simulink model "PROVA__14_10"  (R2020b)
settings: Solver=FixedStepDiscrete  StartTime=0.0  StopTime=Inf  FixedStep=0.02  RelTol=1e-3  EnableMultiTasking=on
undefined symbols (not defined in the file or in its folder): attuatore_Amax, attuatore_Amin, attuatore_Emax, attuatore_Emin, attuatore_Rmax, attuatore_Rmin, attuatore_Tmax, attuatore_Tmin, DiscIntNeverNeededParam, interventoA_05, interventoA_1, interventoE_05, interventoE_1, interventoT, inv_A, inv_comp_h, inv_E, inv_R, inv_T, K_AW_B_AP_quota, K_AW_B_becc, K_AW_B_imb, K_AW_B_roll, K_imb_inv, Kd_h_app, Kd_h_flare, Ki_AP_quota_select, Ki_AP_rotta, Ki_AP_vel, Ki_becch, Ki_h_app, Ki_h_cruise, Ki_h_flare, Ki_roll, Kp_AP_quota_hold_h, Kp_AP_quota_hold_l, Kp_AP_quota_select, Kp_AP_rotta, Kp_AP_vel, Kp_becch, Kp_comp_h, Kp_h_app_max, Kp_h_app_min, Kp_h_cruise, Kp_h_flare, Kp_imb, Kp_p, Kp_q, Kp_roll, Kp_Rotta_ATO, Newton, phi_max, phi_min, Raphson, safe_phi, safe_V, t_AP, theta_max, theta_min, time_alarm_SAFE ... (+5)
libraries: simulink_extras x34, arduinolib x24, pid_lib x8, simulink x3, dspsigops x3, svdutilitieslib x3, aerolibtransform2sys x2, aerolibtransform2 x2
(part 4 of 7)

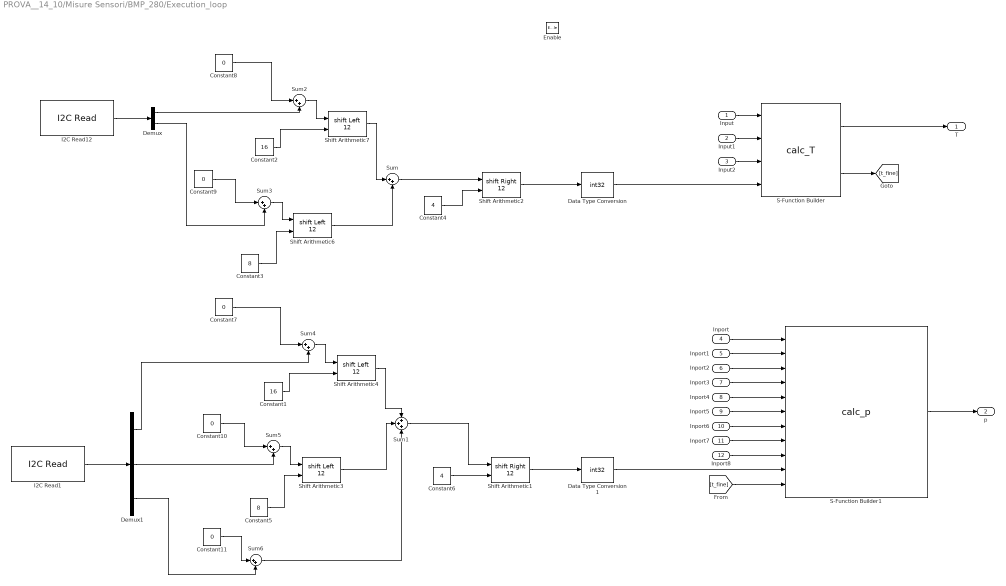
== system PROVA__14_10/Misure Sensori/BMP_280/Execution_loop ==
  Input : Inport
  Input1 : Inport  Port=2
  Input2 : Inport  Port=3
  Inport : Inport  Port=4
  Inport1 : Inport  Port=5
  Inport2 : Inport  Port=6
  Inport3 : Inport  Port=7
  Inport4 : Inport  Port=8
  Inport5 : Inport  Port=9
  Inport6 : Inport  Port=10
  Inport7 : Inport  Port=11
  Inport8 : Inport  Port=12
  Enable : EnablePort
  Constant1 : Constant  Value=16
  Constant{7..11} (5 alike) : Constant  Value=0  OutDataTypeStr=uint32
  Constant2 : Constant  Value=16
  Constant3 : Constant  Value=8
  Constant4 : Constant  Value=4
  Constant5 : Constant  Value=8
  Constant6 : Constant  Value=4
  Data Type Conversion : DataTypeConversion  OutDataTypeStr=int32
  Data Type Conversion1 : DataTypeConversion  OutDataTypeStr=int32
  Demux : Demux  Outputs=2
  Demux1 : Demux  Outputs=3
  I2C Read1 : arduinolib/I2C Read  Priority=2  I2CModule=0  Mode=Master  SlaveAddress=hex2dec( '76' )  SlaveByteOrder=BigEndian  Direction=Receiver  RegisterAddressMode=on  RegisterAddress=hex2dec( 'F7' )  SlaveDataType=uint8  DataLength=3  NoAck=off  RepeatedStart=off  OutputStatus=off  blockPlatform=arduino  SampleTime=t_AP
      settings: AttributesFormatString=Priority=%<Priority>  SourceProductBaseCode=ARDUINO
  I2C Read12 : arduinolib/I2C Read  Priority=1  I2CModule=0  Mode=Master  SlaveAddress=hex2dec( '76' )  SlaveByteOrder=BigEndian  Direction=Receiver  RegisterAddressMode=on  RegisterAddress=hex2dec( 'FA' )  SlaveDataType=uint8  DataLength=2  NoAck=off  RepeatedStart=off  OutputStatus=off  blockPlatform=arduino  SampleTime=t_AP
      settings: AttributesFormatString=Priority=%<Priority>  SourceProductBaseCode=ARDUINO
  S-Function Builder : S-Function  InitFcn=try, set_param(gcb,'FunctionName','calc_T'), end  FunctionName=calc_T  SFunctionModules=calc_T_wrapper  SFunctionDeploymentMode=off  EnableBusSupport=off  mask(S-Function Builder){}
      mask help: Simulink:masks:SFunctionBuilder_MD
      mask init: same as PROVA__14_10/AIR RX/S-Function Builder
      settings: CopyFcn=set_param(gcbh,'LinkStatus','none')  PreSaveFcn=try, set_param(gcb,'FunctionName','calc_T'), end  OpenFcn=sfunctionwizard(gcbh)
      mask Display: plot(val(:,1),val(:,2)),disp(sys), port_label('input',1,'dig_T1'), port_label('input',2,'dig_T2'), port_label('input',3,'dig_T3'), port_label('input',4,'adc_T'), port_label('output',1,'T'), port_label('output',2,'t_fine')
  S-Function Builder1 : S-Function  InitFcn=try, set_param(gcb,'FunctionName','calc_p'), end  FunctionName=calc_p  SFunctionModules=calc_p_wrapper  SFunctionDeploymentMode=off  EnableBusSupport=off  mask(S-Function Builder){}
      mask help: Simulink:masks:SFunctionBuilder_MD
      mask init: same as PROVA__14_10/AIR RX/S-Function Builder
      settings: CopyFcn=set_param(gcbh,'LinkStatus','none')  PreSaveFcn=try, set_param(gcb,'FunctionName','calc_p'), end  OpenFcn=sfunctionwizard(gcbh)
      mask Display: plot(val(:,1),val(:,2)),disp(sys), port_label('input',1,'dig_p1'), port_label('input',2,'dig_p2'), port_label('input',3,'dig_p3'), port_label('input',4,'dig_p4'), port_label('input',5,'dig_p5'), port_label('input',6,'dig_p6'), port_label('input',7,'dig_p7'), port_label('input',8,'dig_p8'), port_label('input',9,'dig_p9'), port_label('input',10,'adc_P'), port_label('input',11,'t_fine'), port_label('output',1,'p')
  Shift Arithmetic1 : ArithShift  BitShiftNumberSource=Input port  BitShiftNumber=12  BitShiftDirection=Right
      settings: InputPortMap=u0,p1
  Shift Arithmetic2 : ArithShift  BitShiftNumberSource=Input port  BitShiftNumber=12  BitShiftDirection=Right
      settings: InputPortMap=u0,p1
  Shift Arithmetic{3..4,6..7} (4 alike) : ArithShift  BitShiftNumberSource=Input port  BitShiftNumber=12  BitShiftDirection=Left
      settings: InputPortMap=u0,p1
  Sum{,2..6} (6 alike) : Sum  Inputs=|++
  Sum1 : Sum  Inputs=+++
  T : Outport  VectorParamsAs1DForOutWhenUnconnected=off
  p : Outport  Port=2  VectorParamsAs1DForOutWhenUnconnected=off
  wires:
  Shift Arithmetic2/1 -> Data Type Conversion/1
  Constant4/1 -> Shift Arithmetic2/2
  S-Function Builder/1 -> T/1
  Input2/1 -> S-Function Builder/3
  Input1/1 -> S-Function Builder/2
  Input/1 -> S-Function Builder/1
  Constant3/1 -> Shift Arithmetic6/2
  Constant2/1 -> Shift Arithmetic7/2
  Shift Arithmetic7/1 -> Sum/1
  Shift Arithmetic6/1 -> Sum/2
  Sum/1 -> Shift Arithmetic2/1
  Sum2/1 -> Shift Arithmetic7/1
  Constant8/1 -> Sum2/1
  Constant9/1 -> Sum3/1
  Demux/2 -> Sum3/2
  Sum3/1 -> Shift Arithmetic6/1
  Data Type Conversion/1 -> S-Function Builder/4
  Shift Arithmetic4/1 -> Sum1/1
  Constant5/1 -> Shift Arithmetic3/2
  Shift Arithmetic1/1 -> Data Type Conversion1/1
  Constant1/1 -> Shift Arithmetic4/2
  Constant6/1 -> Shift Arithmetic1/2
  Sum1/1 -> Shift Arithmetic1/1
  Constant7/1 -> Sum4/1
  S-Function Builder1/1 -> p/1
  Sum5/1 -> Shift Arithmetic3/1
  Constant10/1 -> Sum5/1
  Demux1/2 -> Sum5/2
  Shift Arithmetic3/1 -> Sum1/2
  Sum4/1 -> Shift Arithmetic4/1
  Constant11/1 -> Sum6/1
  Demux1/3 -> Sum6/2
  Sum6/1 -> Sum1/3
  Data Type Conversion1/1 -> S-Function Builder1/10
  Inport/1 -> S-Function Builder1/1
  Inport1/1 -> S-Function Builder1/2
  Inport2/1 -> S-Function Builder1/3
  Inport3/1 -> S-Function Builder1/4
  Inport4/1 -> S-Function Builder1/5
  Inport5/1 -> S-Function Builder1/6
  Inport6/1 -> S-Function Builder1/7
  Inport7/1 -> S-Function Builder1/8
  Inport8/1 -> S-Function Builder1/9
  S-Function Builder/2 -> [t_fine]
  [t_fine] -> S-Function Builder1/11
  I2C Read12/1 -> Demux/1
  Demux/1 -> Sum2/2
  I2C Read1/1 -> Demux1/1
  Demux1/1 -> Sum4/2

== system PROVA__14_10/Misure Sensori/BMP_280/One_time_initialization ==
  Enable : EnablePort
  Bitwise Operator1 : simulink/Logic and Bit Operations/Bitwise Operator  logicop=AND  UseBitMask=on  BitMask=hex2dec('FF')  BitMaskRealWorld=Stored Integer
  Byte Unpack : svdutilitieslib/Byte Unpack  dimensions={[8]}  datatypes={'uint16'}  byteAlign=1  blockPlatform=arduinoert
      settings: SourceProductBaseCode=ANDROID,ARDUINO,ML_ARDUINO,ECCORTEXA,ECCORTEXR,SC_BEAGLEBONE_BLUE,EC_FREEDOM_BOARD,EC_FRDM_K64F,INTEL_BLOCKSET,JETSONCPU,MICROBIT,NUCLEO,NVIDIA,PX4AUTOPILOTS,RASPPIIO,STMICRODIS,TIC2000,XILINX_BLOCKSET
  Constant1 : Constant  Value=hex2dec('0')  OutDataTypeStr=uint8  SampleTime=-1
  Constant4 : Constant  Value=hex2dec('2F')  OutDataTypeStr=uint8  SampleTime=-1
  Data Type Conversion10 : DataTypeConversion  OutDataTypeStr=uint8
  Data Type Conversion11 : DataTypeConversion  OutDataTypeStr=uint8
  I2C Read : arduinolib/I2C Read  Priority=1  I2CModule=0  Mode=Master  SlaveAddress=hex2dec( '76' )  SlaveByteOrder=LittleEndian  Direction=Receiver  RegisterAddressMode=on  RegisterAddress=hex2dec( '88' )  SlaveDataType=uint16  DataLength=1  NoAck=off  RepeatedStart=off  OutputStatus=off  blockPlatform=arduino  SampleTime=t_AP
      settings: AttributesFormatString=Priority=%<Priority>  SourceProductBaseCode=ARDUINO
  I2C Read1 : arduinolib/I2C Read  Priority=2  I2CModule=0  Mode=Master  SlaveAddress=hex2dec( '76' )  SlaveByteOrder=LittleEndian  Direction=Receiver  RegisterAddressMode=on  RegisterAddress=hex2dec( '8A' )  SlaveDataType=int16  DataLength=1  NoAck=off  RepeatedStart=off  OutputStatus=off  blockPlatform=arduino  SampleTime=t_AP
      settings: AttributesFormatString=Priority=%<Priority>  SourceProductBaseCode=ARDUINO
  I2C Read10 : arduinolib/I2C Read  Priority=11  I2CModule=0  Mode=Master  SlaveAddress=hex2dec( '76' )  SlaveByteOrder=LittleEndian  Direction=Receiver  RegisterAddressMode=on  RegisterAddress=hex2dec( '9C' )  SlaveDataType=int16  DataLength=1  NoAck=off  RepeatedStart=off  OutputStatus=off  blockPlatform=arduino  SampleTime=t_AP
      settings: AttributesFormatString=Priority=%<Priority>  SourceProductBaseCode=ARDUINO
  I2C Read11 : arduinolib/I2C Read  Priority=12  I2CModule=0  Mode=Master  SlaveAddress=hex2dec( '76' )  SlaveByteOrder=LittleEndian  Direction=Receiver  RegisterAddressMode=on  RegisterAddress=hex2dec( '9E' )  SlaveDataType=int16  DataLength=1  NoAck=off  RepeatedStart=off  OutputStatus=off  blockPlatform=arduino  SampleTime=t_AP
      settings: AttributesFormatString=Priority=%<Priority>  SourceProductBaseCode=ARDUINO
  I2C Read12 : arduinolib/I2C Read  Priority=16  I2CModule=0  Mode=Master  SlaveAddress=hex2dec( '50' )  SlaveByteOrder=BigEndian  Direction=Receiver  RegisterAddressMode=off  RegisterAddress=0  SlaveDataType=uint8  DataLength=16  NoAck=off  RepeatedStart=off  OutputStatus=off  blockPlatform=ARDUINO  SampleTime=0.02
      settings: AttributesFormatString=Priority=%<Priority>  SourceProductBaseCode=ARDUINO
  I2C Read2 : arduinolib/I2C Read  Priority=3  I2CModule=0  Mode=Master  SlaveAddress=hex2dec( '76' )  SlaveByteOrder=LittleEndian  Direction=Receiver  RegisterAddressMode=on  RegisterAddress=hex2dec( '8C' )  SlaveDataType=int16  DataLength=1  NoAck=off  RepeatedStart=off  OutputStatus=off  blockPlatform=arduino  SampleTime=t_AP
      settings: AttributesFormatString=Priority=%<Priority>  SourceProductBaseCode=ARDUINO
  I2C Read3 : arduinolib/I2C Read  Priority=4  I2CModule=0  Mode=Master  SlaveAddress=hex2dec( '76' )  SlaveByteOrder=LittleEndian  Direction=Receiver  RegisterAddressMode=on  RegisterAddress=hex2dec( '8E' )  SlaveDataType=uint16  DataLength=1  NoAck=off  RepeatedStart=off  OutputStatus=off  blockPlatform=arduino  SampleTime=t_AP
      settings: AttributesFormatString=Priority=%<Priority>  SourceProductBaseCode=ARDUINO
  I2C Read4 : arduinolib/I2C Read  Priority=5  I2CModule=0  Mode=Master  SlaveAddress=hex2dec( '76' )  SlaveByteOrder=LittleEndian  Direction=Receiver  RegisterAddressMode=on  RegisterAddress=hex2dec( '90' )  SlaveDataType=int16  DataLength=1  NoAck=off  RepeatedStart=off  OutputStatus=off  blockPlatform=arduino  SampleTime=t_AP
      settings: AttributesFormatString=Priority=%<Priority>  SourceProductBaseCode=ARDUINO
  I2C Read5 : arduinolib/I2C Read  Priority=6  I2CModule=0  Mode=Master  SlaveAddress=hex2dec( '76' )  SlaveByteOrder=LittleEndian  Direction=Receiver  RegisterAddressMode=on  RegisterAddress=hex2dec( '92' )  SlaveDataType=int16  DataLength=1  NoAck=off  RepeatedStart=off  OutputStatus=off  blockPlatform=arduino  SampleTime=t_AP
      settings: AttributesFormatString=Priority=%<Priority>  SourceProductBaseCode=ARDUINO
  I2C Read6 : arduinolib/I2C Read  Priority=7  I2CModule=0  Mode=Master  SlaveAddress=hex2dec( '76' )  SlaveByteOrder=LittleEndian  Direction=Receiver  RegisterAddressMode=on  RegisterAddress=hex2dec( '94' )  SlaveDataType=int16  DataLength=1  NoAck=off  RepeatedStart=off  OutputStatus=off  blockPlatform=arduino  SampleTime=t_AP
      settings: AttributesFormatString=Priority=%<Priority>  SourceProductBaseCode=ARDUINO
  I2C Read7 : arduinolib/I2C Read  Priority=8  I2CModule=0  Mode=Master  SlaveAddress=hex2dec( '76' )  SlaveByteOrder=LittleEndian  Direction=Receiver  RegisterAddressMode=on  RegisterAddress=hex2dec( '96' )  SlaveDataType=int16  DataLength=1  NoAck=off  RepeatedStart=off  OutputStatus=off  blockPlatform=arduino  SampleTime=t_AP
      settings: AttributesFormatString=Priority=%<Priority>  SourceProductBaseCode=ARDUINO
  I2C Read8 : arduinolib/I2C Read  Priority=9  I2CModule=0  Mode=Master  SlaveAddress=hex2dec( '76' )  SlaveByteOrder=LittleEndian  Direction=Receiver  RegisterAddressMode=on  RegisterAddress=hex2dec( '98' )  SlaveDataType=int16  DataLength=1  NoAck=off  RepeatedStart=off  OutputStatus=off  blockPlatform=arduino  SampleTime=t_AP
      settings: AttributesFormatString=Priority=%<Priority>  SourceProductBaseCode=ARDUINO
  I2C Read9 : arduinolib/I2C Read  Priority=10  I2CModule=0  Mode=Master  SlaveAddress=hex2dec( '76' )  SlaveByteOrder=LittleEndian  Direction=Receiver  RegisterAddressMode=on  RegisterAddress=hex2dec( '9A' )  SlaveDataType=int16  DataLength=1  NoAck=off  RepeatedStart=off  OutputStatus=off  blockPlatform=arduino  SampleTime=t_AP
      settings: AttributesFormatString=Priority=%<Priority>  SourceProductBaseCode=ARDUINO
  I2C Write1 : arduinolib/I2C Write  Priority=13  I2CModule=0  Mode=Master  SlaveAddress=hex2dec( '76' )  SlaveByteOrder=LittleEndian  Direction=Transmitter  RegisterAddressMode=on  RegisterAddress=hex2dec( 'F4' )  SlaveDataType=uint8  DataLength=1  NoAck=off  RepeatedStart=off  OutputStatus=off  blockPlatform=arduino
      settings: AttributesFormatString=Priority=%<Priority>  SourceProductBaseCode=ARDUINO
  I2C Write2 : arduinolib/I2C Write  Priority=14  I2CModule=0  Mode=Master  SlaveAddress=hex2dec( '76' )  SlaveByteOrder=LittleEndian  Direction=Transmitter  RegisterAddressMode=on  RegisterAddress=hex2dec( 'F5' )  SlaveDataType=uint8  DataLength=1  NoAck=off  RepeatedStart=off  OutputStatus=off  blockPlatform=arduino
      settings: AttributesFormatString=Priority=%<Priority>  SourceProductBaseCode=ARDUINO
  I2C Write3 : arduinolib/I2C Write  Priority=15  I2CModule=0  Mode=Master  SlaveAddress=hex2dec( '50' )  SlaveByteOrder=BigEndian  Direction=Transmitter  RegisterAddressMode=off  RegisterAddress=hex2dec( '0' )  SlaveDataType=uint8  DataLength=1  NoAck=off  RepeatedStart=off  OutputStatus=off  blockPlatform=ARDUINO
      settings: AttributesFormatString=Priority=%<Priority>  SourceProductBaseCode=ARDUINO
  Mux1 : Mux  Inputs=2
  Shift Arithmetic1 : ArithShift  BitShiftNumber=8  BitShiftDirection=Right
  "registro memoria2 " : Constant  Value=0  OutDataTypeStr=uint16  SampleTime=t_AP
  dig_T1 : Outport  VectorParamsAs1DForOutWhenUnconnected=off
  dig_T2 : Outport  Port=2  VectorParamsAs1DForOutWhenUnconnected=off
  dig_T3 : Outport  Port=3  VectorParamsAs1DForOutWhenUnconnected=off
  dig_p1 : Outport  Port=4  VectorParamsAs1DForOutWhenUnconnected=off
  dig_p2 : Outport  Port=5  VectorParamsAs1DForOutWhenUnconnected=off
  dig_p3 : Outport  Port=6  VectorParamsAs1DForOutWhenUnconnected=off
  dig_p4 : Outport  Port=7  VectorParamsAs1DForOutWhenUnconnected=off
  dig_p5 : Outport  Port=8  VectorParamsAs1DForOutWhenUnconnected=off
  dig_p6 : Outport  Port=9  VectorParamsAs1DForOutWhenUnconnected=off
  dig_p7 : Outport  Port=10  VectorParamsAs1DForOutWhenUnconnected=off
  dig_p8 : Outport  Port=11  VectorParamsAs1DForOutWhenUnconnected=off
  dig_p9 : Outport  Port=12  VectorParamsAs1DForOutWhenUnconnected=off
  pwm_max_min : Outport  Port=13  VectorParamsAs1DForOutWhenUnconnected=off
  wires:
  Byte Unpack/1 -> pwm_max_min/1
  Data Type Conversion11/1 -> Mux1/2
  "registro memoria2 "/1 -> Bitwise Operator1/1, Shift Arithmetic1/1
  Bitwise Operator1/1 -> Data Type Conversion11/1
  Mux1/1 -> I2C Write3/1
  Shift Arithmetic1/1 -> Data Type Conversion10/1
  Data Type Conversion10/1 -> Mux1/1
  I2C Read12/1 -> Byte Unpack/1
  Constant1/1 -> I2C Write2/1
  Constant4/1 -> I2C Write1/1
  I2C Read1/1 -> dig_T2/1
  I2C Read3/1 -> dig_p1/1
  I2C Read11/1 -> dig_p9/1
  I2C Read9/1 -> dig_p7/1
  I2C Read2/1 -> dig_T3/1
  I2C Read6/1 -> dig_p4/1
  I2C Read5/1 -> dig_p3/1
  I2C Read/1 -> dig_T1/1
  I2C Read4/1 -> dig_p2/1
  I2C Read10/1 -> dig_p8/1
  I2C Read7/1 -> dig_p5/1
  I2C Read8/1 -> dig_p6/1

== system PROVA__14_10/Misure Sensori/BMP_280/Subsystem ==
  T : Inport
  Cal_alt : Inport  Port=2
  T_01 : Inport  Port=3
  Constant : Constant  Value=15
  NotEqual : RelationalOperator  Operator=~=  OutDataTypeStr=boolean  RndMeth=Simplest
  Subsystem1 : Subsystem
  Switch : Switch  Criteria=u2 > Threshold
  Switch1 : Switch  Criteria=u2 > Threshold
  T_02 : Outport  VectorParamsAs1DForOutWhenUnconnected=off
  Cal_alt2 : Outport  Port=2  VectorParamsAs1DForOutWhenUnconnected=off
  wires:
  T_01/1 -> NotEqual/2, Switch1/1, Switch/3
  Switch1/1 -> T_02/1
  Switch/1 -> Switch1/3
  Constant/1 -> NotEqual/1
  Subsystem1/1(T_0) -> Switch/1, Switch/2
  NotEqual/1 -> Switch1/2
  Cal_alt/1 -> Cal_alt2/1, Subsystem1/Enable
  T/1 -> Subsystem1/1(T)

== system PROVA__14_10/Misure Sensori/GPS_Venus/Subsystem1 ==
  h : Inport
  fix : Inport  Port=2
  Enable : EnablePort
  Constant : Constant
  Constant1 : Constant  Value=2
  Constant2 : Constant  Value=0
  Constant3 : Constant  Value=3
  Equal : RelationalOperator  Operator===  OutDataTypeStr=boolean  RndMeth=Simplest
  Equal1 : RelationalOperator  Operator===  OutDataTypeStr=boolean  RndMeth=Simplest
  Equal2 : RelationalOperator  Operator===  OutDataTypeStr=boolean  RndMeth=Simplest
  OR : Logic  Operator=OR  Inputs=3  IconShape=distinctive  AllPortsSameDT=off  OutDataTypeStr=boolean
  Switch : Switch  Criteria=u2 > Threshold
  h_to_subtract : Outport  VectorParamsAs1DForOutWhenUnconnected=off
  wires:
  Constant/1 -> Equal/2
  Equal/1 -> OR/1
  Constant1/1 -> Equal1/2
  Equal1/1 -> OR/2
  h/1 -> Switch/1
  OR/1 -> Switch/2
  Constant2/1 -> Switch/3
  Switch/1 -> h_to_subtract/1
  Equal2/1 -> OR/3
  Constant3/1 -> Equal2/2
  fix/1 -> Equal2/1, Equal1/1, Equal/1

== system PROVA__14_10/Misure Sensori/GPS_Venus/Subsystem2 ==
  In1 : Inport
  Enable : EnablePort
  Create_message : MATLAB Function  TreatAsAtomicUnit=on
  Subsystem : Subsystem
  Misure_GPS : Outport  VectorParamsAs1DForOutWhenUnconnected=off
  mario : Outport  Port=2  VectorParamsAs1DForOutWhenUnconnected=off
  wires:
  In1/1 -> Create_message/1(byte_pack)
  Create_message/2(messaggio) -> Subsystem/1(In1)
  Create_message/1(status) -> Subsystem/Enable
  Subsystem/1(Outport) -> Misure_GPS/1
  Subsystem/2(mario) -> mario/1

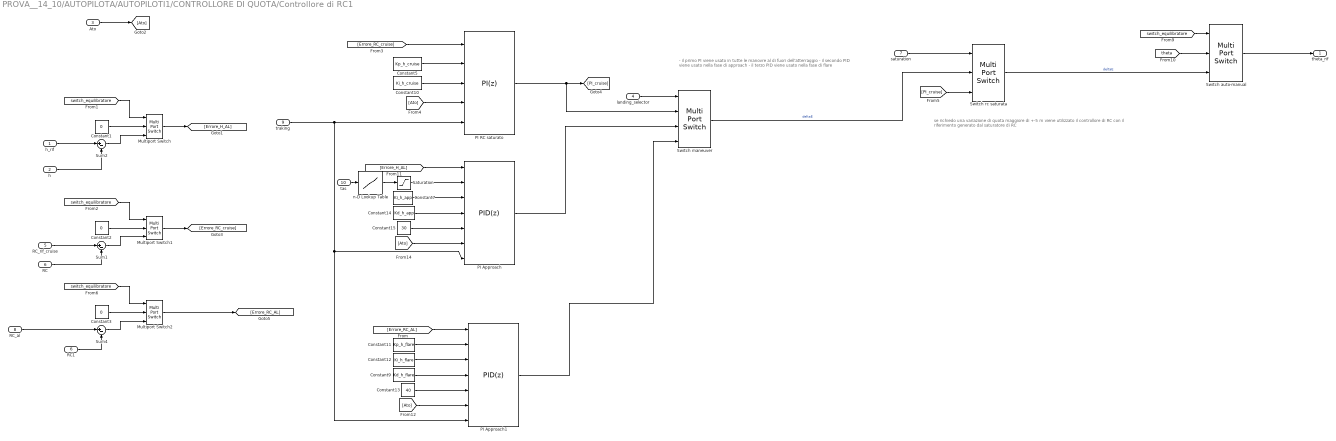
== system PROVA__14_10/AUTOPILOTA/AUTOPILOTI1/CONTROLLORE DI QUOTA/Controllore di RC1 ==
  note: - il primo PI viene usato in tutte le manovre al di fuori dell'atterraggio
      | - il secondo PID viene usato nella fase di approach
      | - il terzo PID viene usato nella fase di flare
  note: se richiedo una variazione di quota maggiore di +-5 m viene utilizzato il controllore di RC
      | con il riferimento generato dal saturatore di RC
  h_rif : Inport
  h : Inport  Port=2
  "Ato " : Inport  Port=3
  landing_selector : Inport  Port=4
  RC_rif_cruise : Inport  Port=5
  RC : Inport  Port=6
  saturation : Inport  Port=7
  "RC_al " : Inport  Port=8
  traking : Inport  Port=9
  tas : Inport  Port=10
  Constant1 : Constant  Value=0  SampleTime=t_AP
  Constant10 : Constant  Value=Ki_h_cruise  SampleTime=t_AP
  Constant11 : Constant  Value=Kp_h_flare  SampleTime=0.02
  Constant12 : Constant  Value=Ki_h_flare  SampleTime=0.02
  Constant13 : Constant  Value=40  SampleTime=0.02
  Constant14 : Constant  Value=Kd_h_app  SampleTime=0.02
  Constant15 : Constant  Value=30  SampleTime=0.02
  Constant2 : Constant  Value=0  SampleTime=t_AP
  Constant3 : Constant  Value=0  SampleTime=t_AP
  Constant5 : Constant  Value=Kp_h_cruise  SampleTime=t_AP
  Constant7 : Constant  Value=Ki_h_app  SampleTime=0.02
  Constant9 : Constant  Value=Kd_h_flare  SampleTime=0.02
  Multiport Switch : MultiPortSwitch  DataPortOrder=Zero-based contiguous  Inputs=2  zeroidx=on
  Multiport Switch1 : MultiPortSwitch  DataPortOrder=Zero-based contiguous  Inputs=2  zeroidx=on
  Multiport Switch2 : MultiPortSwitch  DataPortOrder=Zero-based contiguous  Inputs=2  zeroidx=on
  PI Approach : pid_lib/PID Controller  Controller=PID  Form=Parallel  TimeDomain=Discrete-time  UseExternalTs=off  SampleTime=0.02  IntegratorMethod=Forward Euler  FilterMethod=Forward Euler  ControllerParametersSource=external  P=1  I=1  D=0  UseFilter=on  N=100  TunerSelectOption=Transfer Function Based (PID Tuner App)  InitialConditionSource=internal  InitialConditionForIntegrator=0  InitialConditionForFilter=0  DifferentiatorICPrevScaledInput=0  ExternalReset=rising  TrackingMode=on  Kt=1  LimitOutput=off  SatLimitsSource=internal  UpperSaturationLimit=0.7  LowerSaturationLimit=-0.7  LinearizeAsGain=off  AntiWindupMode=back-calculation  Kb=1  POutMin=[]  POutMax=[]  IOutMin=[]  IOutMax=[]  DOutMin=[]  DOutMax=[]  NOutMin=[]  NOutMax=[]  SumOutMin=[]  SumOutMax=[]  SaturationOutMin=[]  SaturationOutMax=[]  PParamMin=[]  PParamMax=[]  IParamMin=[]  IParamMax=[]  DParamMin=[]  DParamMax=[]  NParamMin=[]  NParamMax=[]  KbParamMin=[]  KbParamMax=[]  KtParamMin=[]  KtParamMax=[]  KbOutMin=[]  KbOutMax=[]  KtOutMin=[]  KtOutMax=[]  IntegratorOutMin=[]  IntegratorOutMax=[]  FilterOutMin=[]  FilterOutMax=[]  SumI1OutMin=[]  SumI1OutMax=[]  SumI2OutMin=[]  SumI2OutMax=[]  SumI3OutMin=[]  SumI3OutMax=[]  SumI4OutMin=[]  SumI4OutMax=[]  SumDOutMin=[]  SumDOutMax=[]  DifferentiatorOutMin=[]  DifferentiatorOutMax=[]  FilterDiffOutCoefMin=[]  FilterDiffOutCoefMax=[]  ReciprocalOutMin=[]  ReciprocalOutMax=[]  SumDenOutMin=[]  SumDenOutMax=[]  SumNumOutMin=[]  SumNumOutMax=[]  DivideOutMin=[]  DivideOutMax=[]  UdiffTsProdOutMin=[]  UdiffTsProdOutMax=[]  NTsProdOutMin=[]  NTsProdOutMax=[]  UintegralTsProdOutMin=[]  UintegralTsProdOutMax=[]  UngainTsProdOutMin=[]  UngainTsProdOutMax=[]  IntegratorContinuousStateAttributes=''  IntegratorStateMustResolveToSignalObject=off  IntegratorRTWStateStorageClass=Auto  FilterContinuousStateAttributes=''  FilterStateMustResolveToSignalObject=off  FilterRTWStateStorageClass=Auto  ParallelPVariant=ExternalParameters  IdealPVariant=Disabled  IVariant=ExternalParameters  DVariant=ExternalParameters  IntegratorVariant=Discrete  SatVariant=Disabled  AWVariant=Passthrough  PCopyVariant=Disabled  TRVariant=Enabled  FdbkBlocksVariant=Forward  IdealPFdbkVariant=Disabled  SatFdbkVariant=Disabled  DerivativeFilterVariant=ForwardEulerFilter  NVariant=ExternalParameters  NCopyVariant=Disabled  FilterICVariant=InternalICsFilter  IntegratorICVariant=InternalICs  ExternalResetVariant=ExternalReset  TRSumVariant=TrackingMode  SumFdbkVariant=Disabled  SumVariant=Sum_PID  TsampFilterVariant=InternalTs  TsampNgainVariant=Passthrough  TsampIntegralVariant=Passthrough  ExternalSaturationOutDataTypeStr=Inherit: Same as second input
  PI Approach1 : pid_lib/PID Controller  Controller=PID  Form=Parallel  TimeDomain=Discrete-time  UseExternalTs=off  SampleTime=0.02  IntegratorMethod=Forward Euler  FilterMethod=Forward Euler  ControllerParametersSource=external  P=1  I=1  D=0  UseFilter=on  N=100  TunerSelectOption=Transfer Function Based (PID Tuner App)  InitialConditionSource=internal  InitialConditionForIntegrator=0  InitialConditionForFilter=0  DifferentiatorICPrevScaledInput=0  ExternalReset=rising  TrackingMode=on  Kt=1  LimitOutput=off  SatLimitsSource=internal  UpperSaturationLimit=0.7  LowerSaturationLimit=-0.7  LinearizeAsGain=off  AntiWindupMode=back-calculation  Kb=1  POutMin=[]  POutMax=[]  IOutMin=[]  IOutMax=[]  DOutMin=[]  DOutMax=[]  NOutMin=[]  NOutMax=[]  SumOutMin=[]  SumOutMax=[]  SaturationOutMin=[]  SaturationOutMax=[]  PParamMin=[]  PParamMax=[]  IParamMin=[]  IParamMax=[]  DParamMin=[]  DParamMax=[]  NParamMin=[]  NParamMax=[]  KbParamMin=[]  KbParamMax=[]  KtParamMin=[]  KtParamMax=[]  KbOutMin=[]  KbOutMax=[]  KtOutMin=[]  KtOutMax=[]  IntegratorOutMin=[]  IntegratorOutMax=[]  FilterOutMin=[]  FilterOutMax=[]  SumI1OutMin=[]  SumI1OutMax=[]  SumI2OutMin=[]  SumI2OutMax=[]  SumI3OutMin=[]  SumI3OutMax=[]  SumI4OutMin=[]  SumI4OutMax=[]  SumDOutMin=[]  SumDOutMax=[]  DifferentiatorOutMin=[]  DifferentiatorOutMax=[]  FilterDiffOutCoefMin=[]  FilterDiffOutCoefMax=[]  ReciprocalOutMin=[]  ReciprocalOutMax=[]  SumDenOutMin=[]  SumDenOutMax=[]  SumNumOutMin=[]  SumNumOutMax=[]  DivideOutMin=[]  DivideOutMax=[]  UdiffTsProdOutMin=[]  UdiffTsProdOutMax=[]  NTsProdOutMin=[]  NTsProdOutMax=[]  UintegralTsProdOutMin=[]  UintegralTsProdOutMax=[]  UngainTsProdOutMin=[]  UngainTsProdOutMax=[]  IntegratorContinuousStateAttributes=''  IntegratorStateMustResolveToSignalObject=off  IntegratorRTWStateStorageClass=Auto  FilterContinuousStateAttributes=''  FilterStateMustResolveToSignalObject=off  FilterRTWStateStorageClass=Auto  ParallelPVariant=ExternalParameters  IdealPVariant=Disabled  IVariant=ExternalParameters  DVariant=ExternalParameters  IntegratorVariant=Discrete  SatVariant=Disabled  AWVariant=Passthrough  PCopyVariant=Disabled  TRVariant=Enabled  FdbkBlocksVariant=Forward  IdealPFdbkVariant=Disabled  SatFdbkVariant=Disabled  DerivativeFilterVariant=ForwardEulerFilter  NVariant=ExternalParameters  NCopyVariant=Disabled  FilterICVariant=InternalICsFilter  IntegratorICVariant=InternalICs  ExternalResetVariant=ExternalReset  TRSumVariant=TrackingMode  SumFdbkVariant=Disabled  SumVariant=Sum_PID  TsampFilterVariant=InternalTs  TsampNgainVariant=Passthrough  TsampIntegralVariant=Passthrough  ExternalSaturationOutDataTypeStr=Inherit: Same as second input
  PI RC saturato : pid_lib/PID Controller  Controller=PI  Form=Parallel  TimeDomain=Discrete-time  UseExternalTs=off  SampleTime=0.02  IntegratorMethod=Forward Euler  FilterMethod=Forward Euler  ControllerParametersSource=external  P=1  I=1  D=0  UseFilter=on  N=100  TunerSelectOption=Transfer Function Based (PID Tuner App)  InitialConditionSource=internal  InitialConditionForIntegrator=0  InitialConditionForFilter=0  DifferentiatorICPrevScaledInput=0  ExternalReset=rising  TrackingMode=on  Kt=1  LimitOutput=off  SatLimitsSource=internal  UpperSaturationLimit=0.7  LowerSaturationLimit=-0.7  LinearizeAsGain=off  AntiWindupMode=back-calculation  Kb=1  POutMin=[]  POutMax=[]  IOutMin=[]  IOutMax=[]  DOutMin=[]  DOutMax=[]  NOutMin=[]  NOutMax=[]  SumOutMin=[]  SumOutMax=[]  SaturationOutMin=[]  SaturationOutMax=[]  PParamMin=[]  PParamMax=[]  IParamMin=[]  IParamMax=[]  DParamMin=[]  DParamMax=[]  NParamMin=[]  NParamMax=[]  KbParamMin=[]  KbParamMax=[]  KtParamMin=[]  KtParamMax=[]  KbOutMin=[]  KbOutMax=[]  KtOutMin=[]  KtOutMax=[]  IntegratorOutMin=[]  IntegratorOutMax=[]  FilterOutMin=[]  FilterOutMax=[]  SumI1OutMin=[]  SumI1OutMax=[]  SumI2OutMin=[]  SumI2OutMax=[]  SumI3OutMin=[]  SumI3OutMax=[]  SumI4OutMin=[]  SumI4OutMax=[]  SumDOutMin=[]  SumDOutMax=[]  DifferentiatorOutMin=[]  DifferentiatorOutMax=[]  FilterDiffOutCoefMin=[]  FilterDiffOutCoefMax=[]  ReciprocalOutMin=[]  ReciprocalOutMax=[]  SumDenOutMin=[]  SumDenOutMax=[]  SumNumOutMin=[]  SumNumOutMax=[]  DivideOutMin=[]  DivideOutMax=[]  UdiffTsProdOutMin=[]  UdiffTsProdOutMax=[]  NTsProdOutMin=[]  NTsProdOutMax=[]  UintegralTsProdOutMin=[]  UintegralTsProdOutMax=[]  UngainTsProdOutMin=[]  UngainTsProdOutMax=[]  IntegratorContinuousStateAttributes=''  IntegratorStateMustResolveToSignalObject=off  IntegratorRTWStateStorageClass=Auto  FilterContinuousStateAttributes=''  FilterStateMustResolveToSignalObject=off  FilterRTWStateStorageClass=Auto  ParallelPVariant=ExternalParameters  IdealPVariant=Disabled  IVariant=ExternalParameters  DVariant=Disabled  IntegratorVariant=Discrete  SatVariant=Disabled  AWVariant=Passthrough  PCopyVariant=Disabled  TRVariant=Enabled  FdbkBlocksVariant=Forward  IdealPFdbkVariant=Disabled  SatFdbkVariant=Disabled  DerivativeFilterVariant=Disabled  NVariant=Disabled  NCopyVariant=Disabled_SignalSpec  FilterICVariant=Disabled  IntegratorICVariant=InternalICs  ExternalResetVariant=ExternalReset  TRSumVariant=TrackingMode  SumFdbkVariant=Disabled  SumVariant=Sum_PI  TsampFilterVariant=InternalTs  TsampNgainVariant=Passthrough  TsampIntegralVariant=Passthrough  ExternalSaturationOutDataTypeStr=Inherit: Same as second input
  RC1 : InportShadow  Port=6
  Saturation : Saturate  UpperLimit=0.046  LowerLimit=0.01
  Sum1 : Sum  Inputs=|+-
  Sum2 : Sum  Inputs=|+-
  Sum4 : Sum  Inputs=|+-
  Switch auto-manual : MultiPortSwitch  DataPortOrder=Zero-based contiguous  Inputs=2  zeroidx=on
  Switch maneuver : MultiPortSwitch  DataPortOrder=Zero-based contiguous  zeroidx=on
  Switch rc saturata : MultiPortSwitch  DataPortOrder=Zero-based contiguous  Inputs=2  zeroidx=on
  n-D Lookup Table : Lookup_n-D  NumberOfTableDimensions=1  BreakpointsForDimension1="[V_stall*1.2  V_max*0.75]"  Table=[Kp_h_app_max Kp_h_app_min]  RndMeth=Simplest  InputSameDT=on
  theta_rif : Outport  VectorParamsAs1DForOutWhenUnconnected=off
  wires:
  landing_selector/1 -> Switch maneuver/1
  [Ato] -> PI Approach/6
  "Ato "/1 -> [Ato]
  [Errore_H_AL] -> PI Approach/1
  [switch_equilibratore] -> Switch auto-manual/1
  [theta] -> Switch auto-manual/2
  Multiport Switch/1 -> [Errore_H_AL]
  [switch_equilibratore] -> Multiport Switch/1
  Constant1/1 -> Multiport Switch/2
  Sum2/1 -> Multiport Switch/3
  h/1 -> Sum2/2
  h_rif/1 -> Sum2/1
  Saturation/1 -> PI Approach/2
  Constant7/1 -> PI Approach/3
  RC_rif_cruise/1 -> Sum1/1
  Sum1/1 -> Multiport Switch1/3
  Constant2/1 -> Multiport Switch1/2
  Multiport Switch1/1 -> [Errore_RC_cruise]
  [switch_equilibratore] -> Multiport Switch1/1
  Switch maneuver/1 -> Switch rc saturata/2  "deltaE"
  RC/1 -> Sum1/2
  saturation/1 -> Switch rc saturata/1
  Switch rc saturata/1 -> Switch auto-manual/3  "deltaE"
  PI RC saturato/1 -> [PI_cruise], Switch maneuver/2
  Constant5/1 -> PI RC saturato/2
  [Ato] -> PI RC saturato/4
  Constant10/1 -> PI RC saturato/3
  [Errore_RC_cruise] -> PI RC saturato/1
  [PI_cruise] -> Switch rc saturata/3
  "RC_al "/1 -> Sum4/1
  [switch_equilibratore] -> Multiport Switch2/1
  RC1/1 -> Sum4/2
  Multiport Switch2/1 -> [Errore_RC_AL]
  Constant3/1 -> Multiport Switch2/2
  Sum4/1 -> Multiport Switch2/3
  PI Approach/1 -> Switch maneuver/3
  [Errore_RC_AL] -> PI Approach1/1
  Constant11/1 -> PI Approach1/2
  Constant12/1 -> PI Approach1/3
  [Ato] -> PI Approach1/6
  Switch auto-manual/1 -> theta_rif/1
  PI Approach1/1 -> Switch maneuver/4
  traking/1 -> PI Approach1/7, PI Approach/7, PI RC saturato/5
  Constant9/1 -> PI Approach1/4
  Constant13/1 -> PI Approach1/5
  Constant14/1 -> PI Approach/4
  Constant15/1 -> PI Approach/5
  tas/1 -> n-D Lookup Table/1
  n-D Lookup Table/1 -> Saturation/1

== system PROVA__14_10/AUTOPILOTA/AUTOPILOTI1/CONTROLLORE DI QUOTA/Saturazione RC  ==
  V : Inport
  RC : Inport  Port=2
  Constant : Constant  Value=-5  SampleTime=t_AP
  Lookup Table2 : Lookup  InputValues=[15;20;25;30;35;40]  Table=[2;2.5;3;3.5;4;4]
  Saturation Dynamic1 : simulink/Discontinuities/Saturation Dynamic  OutMin=[]  OutMax=[]  OutDataTypeStr=Inherit: Same as second input  OutDataType=fixdt(1, 16)  OutScaling=2^-10  DoSatur=off
  RC_verficata : Outport  VectorParamsAs1DForOutWhenUnconnected=off
  wires:
  V/1 -> Lookup Table2/1
  RC/1 -> Saturation Dynamic1/2
  Lookup Table2/1 -> Saturation Dynamic1/1
  Constant/1 -> Saturation Dynamic1/3
  Saturation Dynamic1/1 -> RC_verficata/1

== system PROVA__14_10/AUTOPILOTA/AUTOPILOTI1/CONTROLLORE DI ROTTA/ATO ==
  In1 : Inport
  In2 : Inport  Port=2
  In3 : Inport  Port=3
  In4 : Inport  Port=4
  Constant3 : Constant  Value=Kp_Rotta_ATO
  Constant4 : Constant  Value=0
  Multiport Switch2 : MultiPortSwitch  DataPortOrder=Zero-based contiguous  Inputs=2  zeroidx=on
  Multiport Switch3 : MultiPortSwitch  DataPortOrder=Zero-based contiguous  Inputs=2  zeroidx=on
  Switch3 : Switch  Criteria=u2 > Threshold  Threshold=2
  Switch4 : Switch  Criteria=u2 > Threshold  Threshold=2
  Out1 : Outport  VectorParamsAs1DForOutWhenUnconnected=off
  Out2 : Outport  Port=2  VectorParamsAs1DForOutWhenUnconnected=off
  wires:
  Switch3/1 -> Out1/1
  Constant4/1 -> Multiport Switch3/3
  In1/1 -> Switch3/1, Multiport Switch2/2
  [Switch_ATO] -> Multiport Switch3/1
  [Alt] -> Switch3/2
  Multiport Switch2/1 -> Switch3/3
  [Alt] -> Switch4/2
  [Switch_ATO] -> Multiport Switch2/1
  In4/1 -> Switch4/1, Multiport Switch3/2
  Constant3/1 -> Multiport Switch2/3
  Switch4/1 -> Out2/1
  In2/1 -> [Switch_ATO]
  In3/1 -> [Alt]
  Multiport Switch3/1 -> Switch4/3

== system PROVA__14_10/AUTOPILOTA/AUTOPILOTI1/CONTROLLORE DI ROTTA/calcolo errore Psi  ==
  psi_ref (°) : Inport
  psi (rad) : Inport  Port=2
  Constant : Constant  Value=360  SampleTime=t_AP
  Constant1 : Constant  Value=360  SampleTime=t_AP
  Constant2 : Constant  Value=360  SampleTime=t_AP
  Degrees to Radians : simulink_extras/Transformations/Degrees to Radians
  Math Function : Math  Operator=mod  SignedPower=on  SaturateOnIntegerOverflow=on
  Radians to Degrees : simulink_extras/Transformations/Radians to Degrees
  Sum : Sum  Inputs=|+-
  Sum1 : Sum  Inputs=|+-
  Sum2 : Sum  Inputs=|++
  Switch : Switch  Threshold=180
  Switch1 : Switch  Threshold=-180
  psi_err : Outport  VectorParamsAs1DForOutWhenUnconnected=off
  wires:
  Radians to Degrees/1 -> Math Function/1
  Degrees to Radians/1 -> psi_err/1
  Switch1/1 -> Degrees to Radians/1
  Sum2/1 -> Switch1/3
  Constant2/1 -> Sum2/2
  Switch/1 -> Switch1/1
  Sum/1 -> Sum2/1, Switch1/2, Switch/3, Switch/2, Sum1/1
  Constant1/1 -> Sum1/2
  Sum1/1 -> Switch/1
  Math Function/1 -> Sum/2
  Constant/1 -> Math Function/2
  psi (rad)/1 -> Radians to Degrees/1
  psi_ref (°)/1 -> Sum/1

== system PROVA__14_10/AUTOPILOTA/AUTOPILOTI1/CONTROLLORE DI VELOCITA'/throttle - landing ==
  AL : Inport
  In2 : Inport  Port=2
  Alt : Inport  Port=3
  Constant3 : Constant  Value=0
  Enabled Subsystem : Subsystem  TreatAsAtomicUnit=on
  Hit Crossing : HitCross  HitCrossingOffset=0.3  HitCrossingDirection=falling
  Switch : Switch  Criteria=u2 > Threshold
  throttle - landing : MultiPortSwitch  DataPortOrder=Zero-based contiguous  Inputs=2  zeroidx=on
  Out1 : Outport  VectorParamsAs1DForOutWhenUnconnected=off
  wires:
  Switch/1 -> throttle - landing/3
  throttle - landing/1 -> Out1/1
  AL/1 -> throttle - landing/1
  Alt/1 -> Hit Crossing/1
  In2/1 -> Switch/1, throttle - landing/2
  Constant3/1 -> Switch/3
  Hit Crossing/1 -> Enabled Subsystem/Trigger
  Enabled Subsystem/1(Out1) -> Switch/2

== system PROVA__14_10/AUTOPILOTA/CONTROLLI INTERNI E SWITCH1/Controllore PID/elevator - landing ==
  In1 : Inport
  Tas : Inport  Port=2
  AL : Inport  Port=3
  Constant5 : Constant  Value=0
  Multiport Switch2 : MultiPortSwitch  DataPortOrder=Zero-based contiguous  Inputs=2  zeroidx=on
  Switch1 : Switch  Threshold=16
  Out1 : Outport  VectorParamsAs1DForOutWhenUnconnected=off
  wires:
  Multiport Switch2/1 -> Out1/1
  Tas/1 -> Switch1/2
  In1/1 -> Multiport Switch2/2, Switch1/1
  AL/1 -> Multiport Switch2/1
  Constant5/1 -> Switch1/3
  Switch1/1 -> Multiport Switch2/3

== system PROVA__14_10/AUTOPILOTA/CONTROLLI INTERNI E SWITCH1/Controllore PID/elevator - takeoff ==
  In1 : Inport
  Fase_ATO : Inport  Port=2
  ATO : Inport  Port=3
  eq_rot : Inport  Port=4
  Degrees to Radians : simulink_extras/Transformations/Degrees to Radians
  Multiport Switch1 : MultiPortSwitch  DataPortOrder=Zero-based contiguous  Inputs=5  zeroidx=on
  Multiport Switch2 : MultiPortSwitch  DataPortOrder=Zero-based contiguous  Inputs=2  zeroidx=on
  Out1 : Outport  VectorParamsAs1DForOutWhenUnconnected=off
  wires:
  ATO/1 -> Multiport Switch2/1
  In1/1 -> Multiport Switch1/6, Multiport Switch1/5, Multiport Switch2/2
  Multiport Switch2/1 -> Out1/1
  Multiport Switch1/1 -> Multiport Switch2/3
  Fase_ATO/1 -> Multiport Switch1/1
  eq_rot/1 -> Degrees to Radians/1
  Degrees to Radians/1 -> Multiport Switch1/4, Multiport Switch1/3, Multiport Switch1/2

== system PROVA__14_10/AUTOPILOTA/GESTIONE AUTOPILOTI1/Interruttore_Intervento/Enabled Subsystem ==
  Time : Inport
  Enable : EnablePort
  Constant1 : Constant  Value=0
  Constant2 : Constant
  Switch : Switch  Criteria=u2 > Threshold  Threshold=2
  1/0 : Outport  VectorParamsAs1DForOutWhenUnconnected=off
  wires:
  Time/1 -> Switch/2
  Constant1/1 -> Switch/1
  Constant2/1 -> Switch/3
  Switch/1 -> 1/0/1

== system PROVA__14_10/AUTOPILOTA/GESTIONE AUTOPILOTI1/Interruttore_Intervento/Resettable Subsystem ==
  Reset : ResetPort  DisableCoverage=on
  CLOCK : Subsystem
  Time : Outport  VectorParamsAs1DForOutWhenUnconnected=off
  wires:
  CLOCK/1(Time) -> Time/1

== system PROVA__14_10/AUTOPILOTA/GESTIONE AUTOPILOTI1/Interruttore_Safe/Enabled Subsystem ==
  Time : Inport
  Enable : EnablePort
  Constant1 : Constant  Value=0
  Constant2 : Constant
  Switch : Switch  Criteria=u2 > Threshold  Threshold=2
  1/0 : Outport  VectorParamsAs1DForOutWhenUnconnected=off
  wires:
  Time/1 -> Switch/2
  Constant1/1 -> Switch/1
  Constant2/1 -> Switch/3
  Switch/1 -> 1/0/1

== system PROVA__14_10/AUTOPILOTA/GESTIONE AUTOPILOTI1/Interruttore_Safe/Resettable Subsystem ==
  Reset : ResetPort  DisableCoverage=on
  CLOCK : Subsystem
  Time : Outport  VectorParamsAs1DForOutWhenUnconnected=off
  wires:
  CLOCK/1(Time) -> Time/1

== system PROVA__14_10/AUTOPILOTA/GESTIONE AUTOPILOTI1/Intervento Manager/Alarm_Timing_0.5sec ==
  Intervento_IN : Inport
  "Enabled " : Subsystem  TreatAsAtomicUnit=on
  Resettable Subsystem : Subsystem  TreatAsAtomicUnit=on
  Alarm : Outport  VectorParamsAs1DForOutWhenUnconnected=off
  wires:
  Intervento_IN/1 -> Resettable Subsystem/Reset, "Enabled "/Enable
  Resettable Subsystem/1(Time) -> "Enabled "/1("Time ")
  "Enabled "/1(Alarm_Int) -> Alarm/1

== system PROVA__14_10/AUTOPILOTA/GESTIONE AUTOPILOTI1/Intervento Manager/Alarm_Timing_1sec ==
  Intervento_IN : Inport
  "Enabled " : Subsystem  TreatAsAtomicUnit=on
  Resettable Subsystem : Subsystem  TreatAsAtomicUnit=on
  Alarm : Outport  VectorParamsAs1DForOutWhenUnconnected=off
  wires:
  Intervento_IN/1 -> Resettable Subsystem/Reset, "Enabled "/Enable
  Resettable Subsystem/1(Time) -> "Enabled "/1("Time ")
  "Enabled "/1(Alarm_Int) -> Alarm/1

== system PROVA__14_10/AUTOPILOTA/GESTIONE AUTOPILOTI1/Safe Manager/Alarm_Timing ==
  Alarm_IN : Inport
  "Enabled " : Subsystem  TreatAsAtomicUnit=on
  Resettable Subsystem : Subsystem  TreatAsAtomicUnit=on
  Alarm : Outport  VectorParamsAs1DForOutWhenUnconnected=off
  wires:
  Alarm_IN/1 -> Resettable Subsystem/Reset, "Enabled "/Enable
  Resettable Subsystem/1(Time) -> "Enabled "/1("Time ")
  "Enabled "/1(Alarm Safe) -> Alarm/1

== system PROVA__14_10/AUTOPILOTA/Subsystem1/Subsystem1/APPROACH ==
  dist : Inport
  h_g : Inport  Port=2
  x_g : Inport  Port=3
  V_ : Inport  Port=4
  Enable : EnablePort  ShowOutputPort=on
  Abs : Abs
  Atan : Trigonometry  Operator=atan
  Constant1 : Constant  Value=20  SampleTime=0.02
  Constant2 : Constant  SampleTime=0.02
  Constant3 : Constant  SampleTime=0.02
  Constant4 : Constant  Value=0  SampleTime=0.02
  Discrete-Time Integrator : DiscreteIntegrator  gainval=1  ExternalReset=rising  SampleTime=0.02  LimitOutput=on  UpperSaturationLimit=1  LowerSaturationLimit=0  ICPrevOutput=DiscIntNeverNeededParam  ICPrevScaledInput=DiscIntNeverNeededParam
  Divide : Product  Inputs=*/
  Gain : Gain  Gain=-1
  MATLAB Function : MATLAB Function  TreatAsAtomicUnit=on
  Multiply : Product
  Multiply1 : Product
  Mux : Mux
  Sum : Sum  Inputs=|+-
  Sum1 : Sum  Inputs=|+-
  Switch : Switch  Criteria=u2 > Threshold
  x_g0 : Constant  Value=-100  SampleTime=0.02
  h_ref : Outport  VectorParamsAs1DForOutWhenUnconnected=off
  V1 : Outport  Port=2  VectorParamsAs1DForOutWhenUnconnected=off
  flare_data : Outport  Port=3  VectorParamsAs1DForOutWhenUnconnected=off
  landing_abort : Outport  Port=4  VectorParamsAs1DForOutWhenUnconnected=off
  rc_ref_app : Outport  Port=5  VectorParamsAs1DForOutWhenUnconnected=off
  wires:
  Constant1/1 -> V1/1
  h_g/1 -> Divide/1
  Sum/1 -> Divide/2
  x_g/1 -> Sum/1
  Sum1/1 -> Gain/1
  Gain/1 -> Multiply/2
  dist/1 -> Sum1/1
  x_g0/1 -> Sum/2, MATLAB Function/3(xg0), Sum1/2
  Multiply/1 -> h_ref/1
  Mux/1 -> flare_data/1
  MATLAB Function/2(h_f_out) -> Mux/2
  MATLAB Function/1(x_f_out) -> Mux/1
  Abs/1 -> MATLAB Function/2(gamma)
  MATLAB Function/3(k_x_out) -> Mux/3
  MATLAB Function/4(h_c_out) -> Mux/4
  MATLAB Function/5(no_solution) -> landing_abort/1
  Constant2/1 -> Discrete-Time Integrator/1
  Constant3/1 -> Switch/1
  Enable/1 -> Discrete-Time Integrator/2
  Constant4/1 -> Switch/3
  Discrete-Time Integrator/1 -> Switch/2
  Switch/1 -> MATLAB Function/1(reset)
  V_/1 -> Multiply1/1
  Multiply1/1 -> rc_ref_app/1
  Divide/1 -> Multiply1/2, Multiply/1, Atan/1
  Atan/1 -> Abs/1

== system PROVA__14_10/AUTOPILOTA/Subsystem1/Subsystem1/CREAZIONE_WAYPOINT  ==
  Lat_Home : Inport
  Long_Home : Inport  Port=2
  h_Home : Inport  Port=3
  psi_Home : Inport  Port=4
  AUTOLANDING_WAYPOINTS : MATLAB Function  TreatAsAtomicUnit=on
  Constant : Constant  Value=vel_wp1_al
  Constant1 : Constant  Value=vel_wp2_al
  MATLAB Function : MATLAB Function  TreatAsAtomicUnit=on
  Radians to Degrees : simulink_extras/Transformations/Radians to Degrees
  Radians to Degrees1 : simulink_extras/Transformations/Radians to Degrees
  alt waypoint virtuale : Constant  Value=[45 45 45]
  distance waypoints virtuale : Constant  Value=[-1000 -800 2000]
  WP_info : Outport  VectorParamsAs1DForOutWhenUnconnected=off
  WP_param : Outport  Port=2  VectorParamsAs1DForOutWhenUnconnected=off
  wires:
  alt waypoint virtuale/1 -> AUTOLANDING_WAYPOINTS/4(alt)
  distance waypoints virtuale/1 -> MATLAB Function/4(distance)
  Lat_Home/1 -> MATLAB Function/1(lat_ini)
  Long_Home/1 -> MATLAB Function/2(long_ini)
  psi_Home/1 -> MATLAB Function/3(heading)
  h_Home/1 -> AUTOLANDING_WAYPOINTS/3(h_Home)
  MATLAB Function/1(lat_end) -> Radians to Degrees/1
  MATLAB Function/2(long_end) -> Radians to Degrees1/1
  Radians to Degrees/1 -> AUTOLANDING_WAYPOINTS/1(Lat_Home)
  Radians to Degrees1/1 -> AUTOLANDING_WAYPOINTS/2(Long_Home)
  AUTOLANDING_WAYPOINTS/1(WP_info) -> WP_info/1
  AUTOLANDING_WAYPOINTS/2(WP_param) -> WP_param/1
  Constant/1 -> AUTOLANDING_WAYPOINTS/5(vel_wp1_al)
  Constant1/1 -> AUTOLANDING_WAYPOINTS/6(vel_wp2_al)

== system PROVA__14_10/AUTOPILOTA/Subsystem1/Subsystem1/FLARE ==
  x_e : Inport
  flare_data : Inport  Port=2
  V_ : Inport  Port=3
  Enable : EnablePort
  Constant1 : Constant  Value=18  SampleTime=0.02
  Demux : Demux
  Exp : Math  SignedPower=on  SaturateOnIntegerOverflow=on
  Exp1 : Math  SignedPower=on  SaturateOnIntegerOverflow=on
  Gain : Gain  Gain=-1
  Gain1 : Gain  Gain=-1
  Gain2 : Gain  Gain=-1
  MATLAB Function : MATLAB Function  Commented=on  TreatAsAtomicUnit=on
  Multiply{,1..3} (4 alike) : Product
  Multiply4 : Product  Inputs=3
  Sum{,1,3..4} (4 alike) : Sum  Inputs=|+-
  Sum2 : Sum  Inputs=|++
  x_e1 : InportShadow
  Tas_ref1 : Outport  VectorParamsAs1DForOutWhenUnconnected=off
  h_ref : Outport  Port=2  VectorParamsAs1DForOutWhenUnconnected=off
  RC_ref : Outport  Port=3  VectorParamsAs1DForOutWhenUnconnected=off
  wires:
  MATLAB Function/1(rotta) -> ?
  Constant1/1 -> Tas_ref1/1
  x_e/1 -> Sum/1
  Sum/1 -> Multiply/1
  Multiply/1 -> Gain/1
  Gain/1 -> Exp/1
  Exp/1 -> Multiply1/1
  Sum1/1 -> Multiply1/2
  Multiply1/1 -> Sum2/1
  flare_data/1 -> Demux/1
  Sum2/1 -> h_ref/1
  Gain1/1 -> Exp1/1
  Demux/1 -> Sum3/2, Sum/2  "x_f"
  Demux/2 -> Sum4/1, Sum1/1  "h_f"
  x_e1/1 -> Sum3/1
  Exp1/1 -> Multiply3/1
  Gain2/1 -> RC_ref/1
  Demux/4 -> Sum4/2, Sum1/2, Sum2/2  "h_c"
  Multiply2/1 -> Gain1/1
  Sum3/1 -> Multiply2/1
  Demux/3 -> Multiply2/2, Multiply4/3, Multiply/2  "k_x"
  Multiply3/1 -> Gain2/1
  Sum4/1 -> Multiply4/1
  V_/1 -> Multiply4/2
  Multiply4/1 -> Multiply3/2

== system PROVA__14_10/AUTOPILOTA/Subsystem1/Subsystem1/INSEGUIMENTO CENTRO PISTA ==
  y_e : Inport
  psi_home : Inport  Port=2
  Enable : EnablePort
  Gain1 : Gain
  PID Controller : pid_lib/PID Controller  Controller=PI  Form=Parallel  TimeDomain=Discrete-time  UseExternalTs=off  SampleTime=-1  IntegratorMethod=Forward Euler  FilterMethod=Forward Euler  ControllerParametersSource=external  P=1  I=1  D=0  UseFilter=on  N=100  TunerSelectOption=Transfer Function Based (PID Tuner App)  InitialConditionSource=internal  InitialConditionForIntegrator=0  InitialConditionForFilter=0  DifferentiatorICPrevScaledInput=0  ExternalReset=none  TrackingMode=off  Kt=1  LimitOutput=off  SatLimitsSource=internal  UpperSaturationLimit=inf  LowerSaturationLimit=-inf  LinearizeAsGain=on  AntiWindupMode=none  Kb=1  POutMin=[]  POutMax=[]  IOutMin=[]  IOutMax=[]  DOutMin=[]  DOutMax=[]  NOutMin=[]  NOutMax=[]  SumOutMin=[]  SumOutMax=[]  SaturationOutMin=[]  SaturationOutMax=[]  PParamMin=[]  PParamMax=[]  IParamMin=[]  IParamMax=[]  DParamMin=[]  DParamMax=[]  NParamMin=[]  NParamMax=[]  KbParamMin=[]  KbParamMax=[]  KtParamMin=[]  KtParamMax=[]  KbOutMin=[]  KbOutMax=[]  KtOutMin=[]  KtOutMax=[]  IntegratorOutMin=[]  IntegratorOutMax=[]  FilterOutMin=[]  FilterOutMax=[]  SumI1OutMin=[]  SumI1OutMax=[]  SumI2OutMin=[]  SumI2OutMax=[]  SumI3OutMin=[]  SumI3OutMax=[]  SumI4OutMin=[]  SumI4OutMax=[]  SumDOutMin=[]  SumDOutMax=[]  DifferentiatorOutMin=[]  DifferentiatorOutMax=[]  FilterDiffOutCoefMin=[]  FilterDiffOutCoefMax=[]  ReciprocalOutMin=[]  ReciprocalOutMax=[]  SumDenOutMin=[]  SumDenOutMax=[]  SumNumOutMin=[]  SumNumOutMax=[]  DivideOutMin=[]  DivideOutMax=[]  UdiffTsProdOutMin=[]  UdiffTsProdOutMax=[]  NTsProdOutMin=[]  NTsProdOutMax=[]  UintegralTsProdOutMin=[]  UintegralTsProdOutMax=[]  UngainTsProdOutMin=[]  UngainTsProdOutMax=[]  IntegratorContinuousStateAttributes=''  IntegratorStateMustResolveToSignalObject=off  IntegratorRTWStateStorageClass=Auto  FilterContinuousStateAttributes=''  FilterStateMustResolveToSignalObject=off  FilterRTWStateStorageClass=Auto  ParallelPVariant=ExternalParameters  IdealPVariant=Disabled  IVariant=ExternalParameters  DVariant=Disabled  IntegratorVariant=Discrete  SatVariant=Disabled  AWVariant=Passthrough  PCopyVariant=Disabled  TRVariant=Disabled  FdbkBlocksVariant=Forward  IdealPFdbkVariant=Disabled  SatFdbkVariant=Disabled  DerivativeFilterVariant=Disabled  NVariant=Disabled  NCopyVariant=Disabled_SignalSpec  FilterICVariant=Disabled  IntegratorICVariant=InternalICs  ExternalResetVariant=Disabled  TRSumVariant=Passthrough  SumFdbkVariant=Disabled  SumVariant=Sum_PI  TsampFilterVariant=InternalTs  TsampNgainVariant=Passthrough  TsampIntegralVariant=Passthrough  ExternalSaturationOutDataTypeStr=Inherit: Same as second input
  Radians to Degrees2 : simulink_extras/Transformations/Radians to Degrees
  Sum3 : Sum  Inputs=|+-
  psi ref gain : Constant  Value=0.0052  SampleTime=t_AP
  psi ref gain1 : Constant  Value=0.00052  SampleTime=t_AP
  psi_ref_landing : Outport  VectorParamsAs1DForOutWhenUnconnected=off
  wires:
  psi_home/1 -> [psi_home]
  y_e/1 -> Gain1/1
  Gain1/1 -> PID Controller/1
  psi ref gain/1 -> PID Controller/2
  [psi_home] -> Sum3/1
  Sum3/1 -> Radians to Degrees2/1
  Radians to Degrees2/1 -> psi_ref_landing/1
  psi ref gain1/1 -> PID Controller/3
  PID Controller/1 -> Sum3/2

== system PROVA__14_10/AUTOPILOTA/Subsystem1/Subsystem1/LLA to Flat Earth ==
  latlong : Inport
  h : Inport  Port=2
  ground height : Inport  Port=3
  latlong_ref : Inport  Port=4
  psi_ref : Inport  Port=5
  Degrees to Radians : simulink_extras/Transformations/Degrees to Radians
  LatLong wrap : aerolibtransform2sys/LatLong wrap  SystemSampleTime=-1  VariantActivationTime=update diagram  Latency=0  AutoFrameSizeCalculation=off
      settings: SourceProductBaseCode=AE
  LatLong wrap LL0 : aerolibtransform2sys/LatLong wrap  SystemSampleTime=-1  VariantActivationTime=update diagram  Latency=0  AutoFrameSizeCalculation=off
      settings: SourceProductBaseCode=AE
  Mux : Mux  Inputs=3
  Subsystem1 : Subsystem
  Sum : Sum  Inputs=++|
  Sum1 : Sum  Inputs=|+-
  Ze2height : UnaryMinus
  initial_latg : Selector  InputPortWidth=2  IndexOptions=Index vector (dialog)  Indices=[1]  OutputSizes=1
  Xe : Outport  VectorParamsAs1DForOutWhenUnconnected=off
  wires:
  Degrees to Radians/1 -> Subsystem1/1(pos_rad)
  initial_latg/1 -> Subsystem1/2(mu)
  ground height/1 -> Sum/2
  LatLong wrap/1 -> Degrees to Radians/1
  LatLong wrap LL0/1 -> Sum1/2, initial_latg/1
  Sum1/1 -> LatLong wrap/1
  Ze2height/1 -> Mux/3  "Pz"
  Subsystem1/1(Px) -> Mux/1
  Subsystem1/2(Py) -> Mux/2
  Mux/1 -> Xe/1
  latlong_ref/1 -> LatLong wrap LL0/1
  Sum/1 -> Ze2height/1  "alt"
  h/1 -> Sum/1
  psi_ref/1 -> Subsystem1/3(psi_ref)
  latlong/1 -> Sum1/1

== system PROVA__14_10/Misure Sensori/BMP_280/Subsystem/Subsystem1 ==
  T : Inport
  Enable : EnablePort
  T_0 : Outport  VectorParamsAs1DForOutWhenUnconnected=off
  wires:
  T/1 -> T_0/1

== system PROVA__14_10/Misure Sensori/GPS_Venus/Subsystem2/Subsystem ==
  In1 : Inport
  Enable : EnablePort
  Complex to Real-Imag : ComplexToRealImag  Output=Real
  MATLAB Function : MATLAB Function  TreatAsAtomicUnit=on
  Memory : Memory  InheritSampleTime=on
  Mux : Mux  Inputs=9
  Outport : Outport  VectorParamsAs1DForOutWhenUnconnected=off
  mario : Outport  Port=2  VectorParamsAs1DForOutWhenUnconnected=off
  wires:
  MATLAB Function/2(Long) -> Mux/2  "Long"
  Memory/1 -> MATLAB Function/2(out_prec)
  MATLAB Function/8(h_mean_sea) -> Mux/8  "h_mean_sea"
  MATLAB Function/3(V) -> Mux/3  "hor_speed"
  MATLAB Function/1(Lat) -> Mux/1  "Lat"
  Mux/1 -> Complex to Real-Imag/1
  MATLAB Function/9(h_WGS84) -> Mux/9  "h_WGS85"
  MATLAB Function/5(heading) -> Mux/5  "heading"
  MATLAB Function/6(fix_mode) -> Mux/6  "fix_GPS"
  MATLAB Function/4(Magnetic_declination) -> Mux/4
  MATLAB Function/7(n_sat) -> Mux/7
  Complex to Real-Imag/1 -> Memory/1, Outport/1
  In1/1 -> MATLAB Function/1(messaggio)
  MATLAB Function/10(indice_dimario) -> mario/1
